simulink library "libAUVT"  (Simulink 7.6)
settings: Solver=ode45  StartTime=0.0  StopTime=10.0  RelTol=1e-3
undefined symbols (not defined in the file or in its folder): DiscIntNeverNeededParam
libraries: libAUVT x1, simulink x1
settings Model: Creator=auvt  LastModifiedBy=auvt

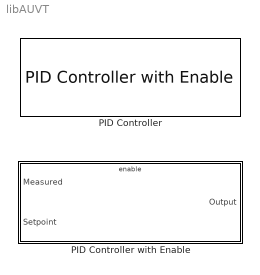
== system libAUVT ==
  PID Controller : libAUVT/PID Controller with Enable  SystemSampleTime=-1  Kp=0  Ki=0  Kd=0
  PID Controller with Enable : Subsystem  mask{Kp=0, Ki=0, Kd=0}
      mask prompts: Kp "Proportional Gain"; Ki "Integral Gain"; Kd "Derivative Gain"
      mask help: Simple PID Controller
      mask TabNameString: Gains,Gains,Gains

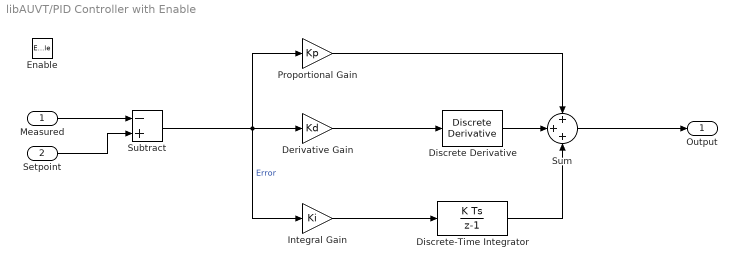
== system libAUVT/PID Controller with Enable ==
  Measured : Inport
  Setpoint : Inport  Port=2
  Enable : EnablePort  StatesWhenEnabling=reset
  Derivative Gain : Gain  Gain=Kd
  Discrete Derivative : simulink/Discrete/Discrete Derivative  SystemSampleTime=-1  gainval=1  ICPrevScaledInput=0.0  OutMin=[]  OutMax=[]  OutDataType=fixdt(1, 16)  OutScaling=2^-10  DoSatur=off
  Discrete-Time Integrator : DiscreteIntegrator  gainval=1  SampleTime=-1  LimitOutput=on  UpperSaturationLimit=15  LowerSaturationLimit=-15  ICPrevOutput=DiscIntNeverNeededParam  ICPrevScaledInput=DiscIntNeverNeededParam
  Integral Gain : Gain  Gain=Ki
  Proportional Gain : Gain  Gain=Kp
  Subtract : Sum  Inputs=-+
  Sum : Sum  Inputs=+++  SaturateOnIntegerOverflow=on  InputSameDT=on  OutDataTypeStr=Inherit: Same as first input
  Output : Outport  OutputWhenDisabled=reset  InitialOutput=0
  wires:
  Sum/1 -> Output/1
  Integral Gain/1 -> Discrete-Time Integrator/1
  Derivative Gain/1 -> Discrete Derivative/1
  Discrete Derivative/1 -> Sum/2
  Proportional Gain/1 -> Sum/1
  Discrete-Time Integrator/1 -> Sum/3
  Setpoint/1 -> Subtract/2
  Measured/1 -> Subtract/1
  Subtract/1 -> Integral Gain/1, Derivative Gain/1, Proportional Gain/1  "Error"
